simulink model "no control"  (R2016a)
settings: Solver=VariableStepAuto  StartTime=0.0  StopTime=inf  FixedStep=0.005  RelTol=1e-3
PreLoadFcn:
  | load('param.mat')
libraries: LibrarySimulinkSAS x5, realtime_pacer_lib x1
settings Model: Creator=M  LastModifiedBy=M

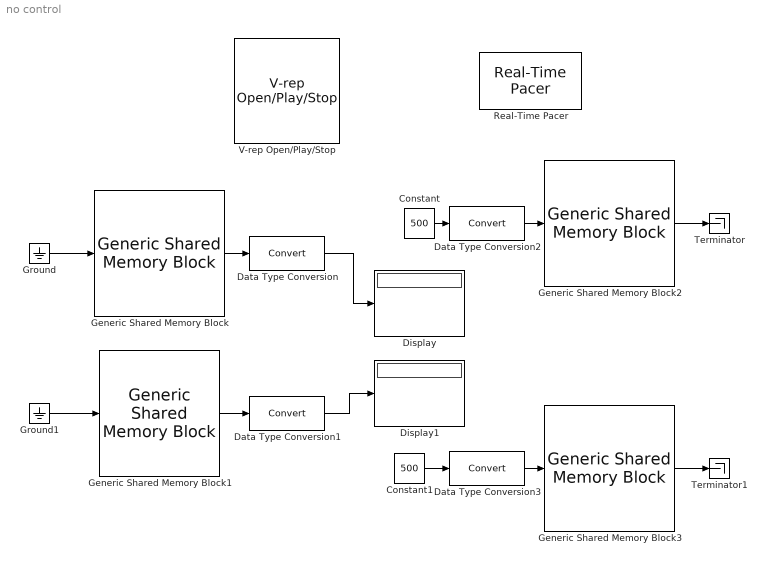
== system no control ==
  Constant : Constant  Value=500
  Constant1 : Constant  Value=500
  Data Type Conversion{,1..3} (4 alike) : DataTypeConversion
  Display : Display
  Display1 : Display
  Generic Shared Memory Block : LibrarySimulinkSAS/Generic Shared Memory Block  nombre='vel_torq_left'  dispositivo=1  vecE=[1]  vecS=[2]  tipoE=['f']  tipoS=['f']  ts=-1
  Generic Shared Memory Block1 : LibrarySimulinkSAS/Generic Shared Memory Block  nombre='vel_torq_right'  dispositivo=2  vecE=[1]  vecS=[2]  tipoE=['f']  tipoS=['f']  ts=-1
  Generic Shared Memory Block2 : LibrarySimulinkSAS/Generic Shared Memory Block  nombre='set_torq_left'  dispositivo=3  vecE=[1]  vecS=[1]  tipoE=['f']  tipoS=['f']  ts=-1
  Generic Shared Memory Block3 : LibrarySimulinkSAS/Generic Shared Memory Block  nombre='set_torq_right'  dispositivo=4  vecE=[1]  vecS=[1]  tipoE=['f']  tipoS=['f']  ts=-1
  Ground : Ground
  Ground1 : Ground
  Real-Time Pacer : realtime_pacer_lib/Real-Time Pacer  simTimePerRealTime=1
  Terminator : Terminator
  Terminator1 : Terminator
  V-rep Open/Play/Stop : LibrarySimulinkSAS/V-rep Open//Play//Stop  scene='cuboidVrep.ttt'
  wires:
  Ground/1 -> Generic Shared Memory Block/1
  Generic Shared Memory Block1/1 -> Data Type Conversion1/1
  Ground1/1 -> Generic Shared Memory Block1/1
  Generic Shared Memory Block2/1 -> Terminator/1
  Generic Shared Memory Block3/1 -> Terminator1/1
  Generic Shared Memory Block/1 -> Data Type Conversion/1
  Data Type Conversion/1 -> Display/1
  Data Type Conversion1/1 -> Display1/1
  Constant/1 -> Data Type Conversion2/1
  Data Type Conversion2/1 -> Generic Shared Memory Block2/1
  Constant1/1 -> Data Type Conversion3/1
  Data Type Conversion3/1 -> Generic Shared Memory Block3/1
